simulink model "Simulation_Problem3"  (R2024a)
settings: Solver=VariableStepAuto  StartTime=0.0  StopTime=10.0  MaxStep=0.001
settings Model: Creator=hp  LastModifiedBy=hp

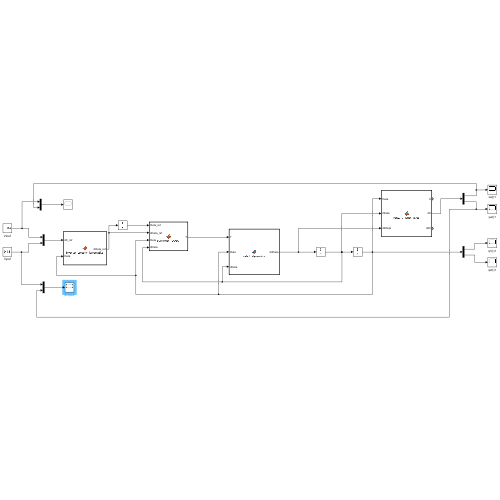
[thumbnail: Simulink's stored preview of the top-level diagram]
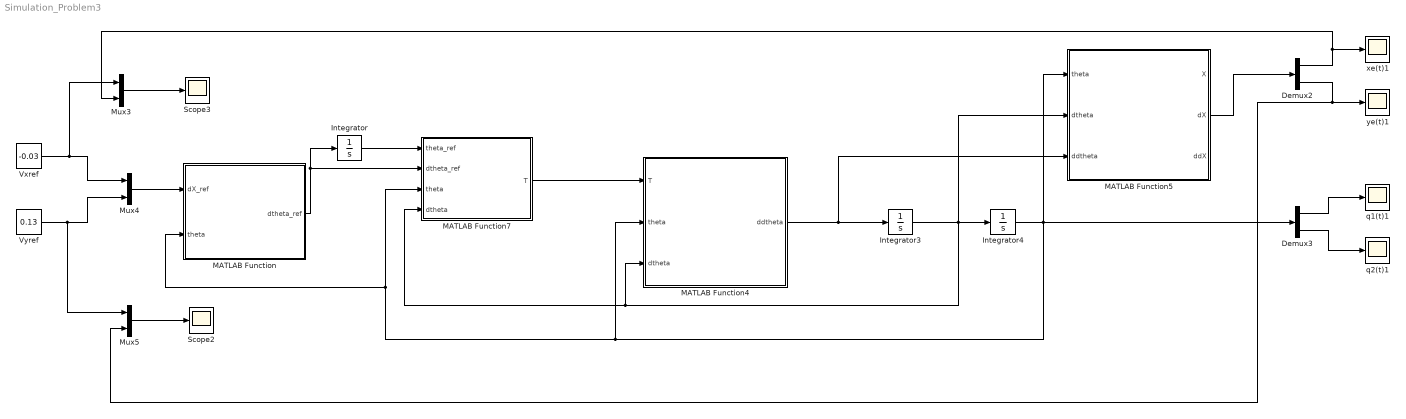
== system Simulation_Problem3 ==
  Demux2 : Demux  Outputs=2
  Demux3 : Demux  Outputs=2
  Integrator : Integrator  InitialCondition=[pi/4; pi/4]
  Integrator3 : Integrator  InitialCondition=[0; 0]
  Integrator4 : Integrator  InitialCondition=[pi/4; pi/4]
  MATLAB Function : MATLAB Function  TreatAsAtomicUnit=on
  MATLAB Function4 : MATLAB Function  TreatAsAtomicUnit=on
  MATLAB Function5 : MATLAB Function  TreatAsAtomicUnit=on
  MATLAB Function7 : MATLAB Function  TreatAsAtomicUnit=on
  Mux3 : Mux  Inputs=2
  Mux4 : Mux  Inputs=2
  Mux5 : Mux  Inputs=2
  Scope2 : Scope
  Scope3 : Scope
  Vxref : Constant  Value=-0.03
  Vyref : Constant  Value=0.13
  q1(t)1 : Scope
  q2(t)1 : Scope
  xe(t)1 : Scope
  ye(t)1 : Scope
  wires:
  Mux5/1 -> Scope2/1
  Demux3/1 -> q1(t)1/1
  Integrator3/1 -> MATLAB Function5/2(dtheta), MATLAB Function7/4(dtheta), MATLAB Function4/3(dtheta), Integrator4/1
  MATLAB Function7/1(T) -> MATLAB Function4/1(T)
  Mux4/1 -> MATLAB Function/1(dX_ref)
  MATLAB Function/1(dtheta_ref) -> Integrator/1, MATLAB Function7/2(dtheta_ref)
  Integrator4/1 -> Demux3/1, MATLAB Function5/1(theta), MATLAB Function7/3(theta), MATLAB Function/2(theta), MATLAB Function4/2(theta)
  Mux3/1 -> Scope3/1
  Vxref/1 -> Mux3/1, Mux4/1
  Demux3/2 -> q2(t)1/1
  Demux2/2 -> Mux5/2, ye(t)1/1
  Demux2/1 -> Mux3/2, xe(t)1/1
  MATLAB Function4/1(ddtheta) -> MATLAB Function5/3(ddtheta), Integrator3/1
  Vyref/1 -> Mux5/1, Mux4/2
  Integrator/1 -> MATLAB Function7/1(theta_ref)
  MATLAB Function5/2(dX) -> Demux2/1

== matlab function Simulation_Problem3/MATLAB Function ==
  data: dX_ref input; dtheta_ref output; theta input
function dtheta_ref = inverse_velocity_kinematics(dX_ref, theta)
% Uç nokta referans hizini (dX_ref), eklem referans hizlarina (dtheta_ref) cevirir.

l1 = 0.83; 
l2 = 0.46;
th1 = theta(1); th2 = theta(2);

% Jacobian Matrisi
J11 = -l1*sin(th1) - l2*sin(th1+th2);
J12 = -l2*sin(th1+th2);
J21 = l1*cos(th1) + l2*cos(th1+th2);
J22 = l2*cos(th1+th2);
J = [J11, J12; J21, J22];

dtheta_ref = J \ dX_ref;
end

== matlab function Simulation_Problem3/MATLAB Function4 ==
  data: T input; ddtheta output; theta input; dtheta input
function ddtheta = robot_dynamics(T, theta, dtheta)
% Problem 1 - Dinamik Model

% Kendi grubumuzun degerlerini garanti olsun diye buraya da yaziyoruz 
% (Simulink'in Workspace'den cekerken hata vermesini engellemek icin)
l1 = 0.83; l2 = 0.46;
r1 = 0.42; r2 = 0.23;
m1 = 0.66; m2 = 0.37;
I1 = 0.03; I2 = 0.02;
g = 9.81;

th1 = theta(1); th2 = theta(2);
dth1 = dtheta(1); dth2 = dtheta(2);
T1 = T(1); T2 = T(2);

% A(theta) Matrisi Parametreleri
a11 = m2*l1^2 + 2*m2*l1*r2*cos(th2) + m1*r1^2 + m2*r2^2 + I1 + I2; 
a12 = m2*r2^2 + l1*m2*r2*cos(th2) + I2; 
a21 = m2*r2^2 + l1*m2*r2*cos(th2) + I2; 
a22 = m2*r2^2 + I2; 
A = [a11, a12; a21, a22]; 

% B(theta, dtheta) Matrisi Parametreleri
b11 = -2*l1*m2*r2*sin(th2)*dth2; 
b12 = -2*l1*m2*r2*sin(th2)*dth1 - 2*l1*m2*r2*sin(th2)*dth2; 
b21 = 2*l1*m2*r2*sin(th2)*dth1; 
b22 = 0; 
B = [b11, b12; b21, b22]; 

% G(theta) Matrisi Parametreleri
g1 = m2*r2*g*cos(th1+th2) + m2*l1*g*cos(th1) + m1*r1*g*cos(th1); 
g2 = m2*r2*g*cos(th1+th2); 
G = [g1; g2]; 

% Tork Vektoru
Tau = [T1; T2];

% Dinamik Denklemin Cozumu
ddtheta = A \ (Tau - B*dtheta - G); 
end

== matlab function Simulation_Problem3/MATLAB Function5 ==
  data: theta input; X output; dtheta input; ddtheta input; dX output; ddX output
function [X, dX, ddX] = forward_kinematics(theta, dtheta, ddtheta)
% Ileri Kinematik ve Jacobian Hesaplamalari
% Problem 1 - Uç Nokta Degerleri

% l1 ve l2 degerleri
l1 = 0.83; 
l2 = 0.46;

th1 = theta(1); th2 = theta(2);
dth1 = dtheta(1); dth2 = dtheta(2);
ddth1 = ddtheta(1); ddth2 = ddtheta(2);

% 1. Konum (X)
xe = l1*cos(th1) + l2*cos(th1+th2);
ye = l1*sin(th1) + l2*sin(th1+th2);
X = [xe; ye];

% 2. Jacobian Matrisi ve Hiz (dX)
J11 = -l1*sin(th1) - l2*sin(th1+th2);
J12 = -l2*sin(th1+th2);
J21 = l1*cos(th1) + l2*cos(th1+th2);
J22 = l2*cos(th1+th2);
J = [J11, J12; J21, J22];

dX = J * [dth1; dth2];

% 3. Jacobian Turevi ve Ivme (ddX)
dJ11 = -l1*cos(th1)*dth1 - l2*cos(th1+th2)*(dth1+dth2);
dJ12 = -l2*cos(th1+th2)*(dth1+dth2);
dJ21 = -l1*sin(th1)*dth1 - l2*sin(th1+th2)*(dth1+dth2);
dJ22 = -l2*sin(th1+th2)*(dth1+dth2);
dJ = [dJ11, dJ12; dJ21, dJ22];

ddX = dJ * [dth1; dth2] + J * [ddth1; ddth2];
end

== matlab function Simulation_Problem3/MATLAB Function7 ==
  data: theta_ref input; dtheta_ref input; T output; theta input; dtheta input
function T = controller_DOob(theta_ref, dtheta_ref, theta, dtheta)
% Problem 2 - Konum Kontrolcusu ve Gozlemci 

% Grubun Degerleri
l1 = 0.83; l2 = 0.46;
r1 = 0.42; r2 = 0.23;
m1 = 0.66; m2 = 0.37;
I1 = 0.03; I2 = 0.02;
g = 9.81;

% PD Kontrol Katsayilari
Kp = 150;
Kd = 30;

th1 = theta(1); th2 = theta(2);
dth1 = dtheta(1); dth2 = dtheta(2);

% 1. Adim: PD Konum Kontrolcusu (Sadece ivme referansi uretir)
ddtheta_ref = Kp * (theta_ref - theta) + Kd * (dtheta_ref - dtheta);

% 2. Adim: Dinamik Model / Gozlemci Kompanzasyonu
a11 = m2*l1^2 + 2*m2*l1*r2*cos(th2) + m1*r1^2 + m2*r2^2 + I1 + I2;
a12 = m2*r2^2 + l1*m2*r2*cos(th2) + I2;
a21 = m2*r2^2 + l1*m2*r2*cos(th2) + I2;
a22 = m2*r2^2 + I2;
A = [a11, a12; a21, a22];

b11 = -2*l1*m2*r2*sin(th2)*dth2;
b12 = -2*l1*m2*r2*sin(th2)*dth1 - 2*l1*m2*r2*sin(th2)*dth2;
b21 = 2*l1*m2*r2*sin(th2)*dth1;
b22 = 0;
B = [b11, b12; b21, b22];

g1 = m2*r2*g*cos(th1+th2) + m2*l1*g*cos(th1) + m1*r1*g*cos(th1);
g2 = m2*r2*g*cos(th1+th2);
G = [g1; g2];

% Motorlara gidecek nihai Tork (T = A*ddtheta_ref + B*dtheta + G)
T = A * ddtheta_ref + B * dtheta + G;
end
